simulink model "servoHbridgePraxisbericht"  (R2015a)
settings: Solver=ode23tb  StartTime=0.0  StopTime=1  MaxStep=0.02  RelTol=1e-4
model workspace (MATLAB code in the model file):
  | m_Kt=1.8; % Torque constant
values from neighbouring files (symbols this model uses):
  A = zeros(SYMPACLEN, SYMPACLEN)    [InputMatFramer.m]    (also in InputMatFramerAbgespeckt.m = zeros(10, 10); OUT_OF_MEMORY.m; TIPS_TRICKS.m = { sqrt(10*(rand(2,10)-0.5)), [sqrt(10*(rand(2,10)-0.5)) sqrt; UngarischeMethode.m = [[1 2 9 8];[3 0 3 2];[7 4 1 4];[4 2 7 7]])
  N = (2^16-1)    (= 65535)    [AD_DA.m]    (also in AFB_polynom_interpol.m = 8; UMTSb.m = 160000)
undefined symbols (not defined in the file or in its folder): sigbuilder_block
libraries: powerlib x19
Description:
  | Copyright 2008-2015 The MathWorks, Inc.
settings Model: CovSFcnEnable=off  Creator=MathWorks  LastModifiedBy=mainster
settings DataIOCC: SignalLoggingSaveFormat=ModelDataLogs
settings OptimizationCC: ExpressionDepthLimit=2147483647  InitFltsAndDblsToZero=on
settings DebuggingCC: SaveWithParameterizedLinksMsg=none  UnderspecifiedInitializationDetection=Classic  MergeDetectMultiDrivingBlocksExec=none  SignalResolutionControl=TryResolveAllWithWarning  MaxConsecutiveZCsMsg=warning  SolverPrmCheckMsg=warning  MultiTaskDSMMsg=warning  MultiTaskCondExecSysMsg=none  FcnCallInpInsideContextMsg=UseLocalSettings  StateNameClashWarn=warning
settings GRTTargetCC: TargetFcnLib=ansi_tfl_tmw.mat  CombineOutputUpdateFcns=off  GRTInterface=on

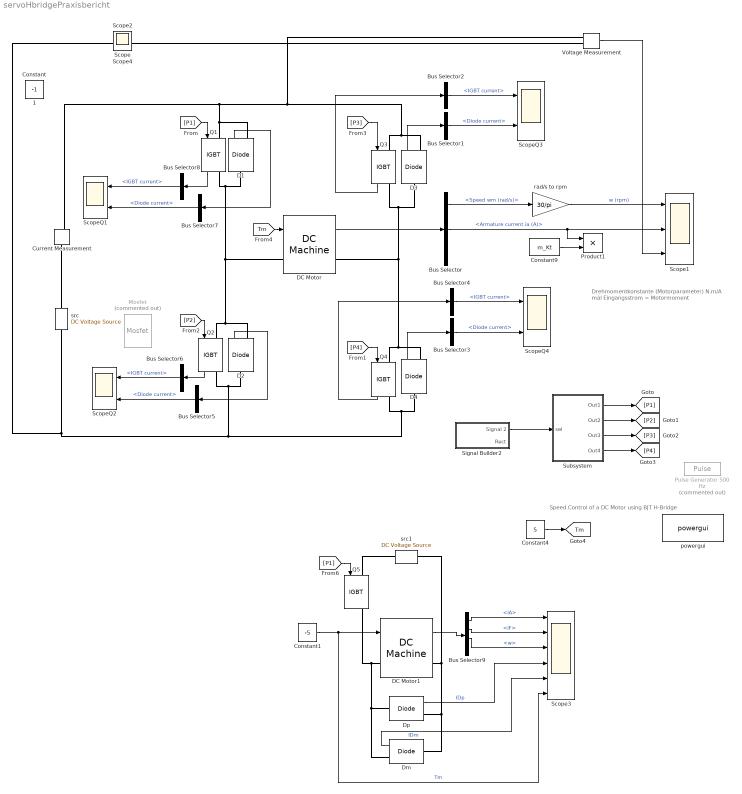
== system servoHbridgePraxisbericht ==
  note: Drehmomentkonstante (Motorparameter) N.m/A
      | mal Eingangsstrom = Motormoment
  note: Speed Control of a DC Motor using BJT H-Bridge
  Bus Selector : BusSelector  OutputSignals=Speed wm (rad/s),Armature current ia (A),Electrical torque Te (n m)
  Bus Selector{1,3,5,7} (4 alike) : BusSelector  OutputSignals=Diode current
  Bus Selector{2,4,6,8} (4 alike) : BusSelector  OutputSignals=IGBT current
  Bus Selector9 : BusSelector  OutputSignals=iA,iF,w,Te
  Constant1 : Constant  Value=-5
  Constant4 : Constant  Value=5
  Constant9 : Constant  Value=m_Kt
  Current Measurement : powerlib/Measurements/Current Measurement  PhasorSimulation=off  OutputType=Complex  PSBequivalent=0
  D{1..4} (4 alike) : powerlib/Power Electronics/Diode  Ron=0.001  Lon=0  Vf=0.8  IC=0  UseSnubber=off  Rs=inf  Cs=0  Measurements=on
  DC Motor : powerlib/Machines/DC Machine  PresetModel=No  MechanicalLoad=Torque TL  FieldType=Permanent magnet  ShowDetailedParameters=on  MeasurementBus=off  RLa=[1 10e-3]  RLf=[281.2 156]  Laf=0.9483  MachineConstant=Torque constant (N.m/A)  Ke=1.8  Kt=m_Kt  J=0.02215  Bm=0.002953  Tf=0.5161  w0=0.001  Ifinit=1.06647707074298  TsPowergui=0  TsBlock=-1
  DC Motor1 : powerlib/Machines/DC Machine  PresetModel=No  MechanicalLoad=Torque TL  FieldType=Permanent magnet  ShowDetailedParameters=on  MeasurementBus=on  RLa=[10 10e-3]  RLf=[281.2 156]  Laf=0.9483  MachineConstant=Torque constant (N.m/A)  Ke=1.8  Kt=m_Kt  J=0.02215  Bm=0.002953  Tf=0.5161  w0=0.001  Ifinit=1  TsPowergui=0  TsBlock=-1
  Dm : powerlib/Power Electronics/Diode  Ron=0.001  Lon=0  Vf=0.8  IC=0  UseSnubber=off  Rs=inf  Cs=0  Measurements=on
  Dp : powerlib/Power Electronics/Diode  Ron=0.001  Lon=0  Vf=0.8  IC=0  UseSnubber=off  Rs=inf  Cs=0  Measurements=on
  Mosfet : powerlib/Power Electronics/Mosfet  Commented=on  Ron=0.1  Lon=0  Rd=0.01  Vfd=.7  IC=0  Rs=1e5  Cs=inf  Measurements=on
  Product1 : Product  RndMeth=Zero
  Pulse Generator 500 Hz : DiscretePulseGenerator  Commented=on  PulseType=Time based  Period=2e-3  PulseWidth=75
  Q{1..5} (5 alike) : powerlib/Power Electronics/IGBT  Ron=0.001  Lon=0  Vf=1  Tf=0  Tt=0  IC=0  Rs=1e5  Cs=inf  Measurements=on
  Scope1 : Scope  NumInputPorts=3
      settings: TimeRange=1  YMin=-100~-10~-20  YMax=100~20~40
  Scope3 : Scope  NumInputPorts=6
      settings: TimeRange=1  YMin=0~-1~-15~-2000~-10~4  YMax=4~1~5~6000~5~6  SaveName=ScopeData7
  ScopeQ{1..4} (4 alike) : Scope  NumInputPorts=2
      ScopeQ1 settings: TimeRange=1  YMin=0~-1  YMax=15~1  SaveName=ScopeData4
      ScopeQ2 settings: TimeRange=1  YMin=0~0  YMax=4~4  SaveName=ScopeData3
      ScopeQ3 settings: TimeRange=1  YMin=0~0  YMax=4~4
      ScopeQ4 settings: TimeRange=1  YMin=0~-1  YMax=15~1  SaveName=ScopeData2
  Signal Builder2 : Subsystem  Tag=STV Subsys  LoadFcn=sigbuilder_block('load');  StartFcn=sigbuilder_block('start');  StopFcn=sigbuilder_block('stop');  ClipboardFcn=sigbuilder_block('clipboard');  mask(Sigbuilder block){}
      mask help: Simulink:masks:SigbuilderBlock_MD
      mask init:
      | if ~strcmp(get_param(bdroot(gcbh),'SimulationStatus'),'stopped') tuvar = sigbuilder_block('maskInit'); end
      settings: CopyFcn=sigbuilder_block('copy');  DeleteFcn=sigbuilder_block('delete');  ModelCloseFcn=sigbuilder_block('modelClose');  PreSaveFcn=sigbuilder_block('preSave');  PauseFcn=sigbuilder_block('pause');  ContinueFcn=sigbuilder_block('continue');  NameChangeFcn=sigbuilder_block('namechange');  OpenFcn=sigbuilder_block('open',[437.6 199.2 550.4 400 ]);  CloseFcn=sigbuilder_block('close');
      mask Display: plot(0, 0, 100, 100,[2, 2, 32, 32, 2], [68, 8, 8, 68, 68],[32, 2], [38, 38], [32, 19, 2],[53, 60, 44], [32, 17, 17, 2],[16, 16, 31, 31]);txt = getActiveGroup(gcbh);text(2, 100, txt,'verticalAlignment', 'top');
  Subsystem : Subsystem
  Voltage Measurement : powerlib/Measurements/Voltage Measurement  PhasorSimulation=off  OutputType=Complex  PSBequivalent=0
  powergui : powerlib/powergui  SimulationMode=Continuous  SolverType=Tustin  SampleTime=20e-6  frequency=60  SPID=on  DisableSnubberDevices=on  DisableRonSwitches=off  DisableVfSwitches=off  SwTol=0  DisplayEquations=off  Interpol=off  methode=off  Ts=0  FunctionMessages=off  echomessages=off  HookPort=off  EnableUseOfTLC=off  x0status=blocks  frequencyindice=0  Pbase=100e6  ErrMax=1e-4  Iterations=50  UnitsV=kV  UnitsW=MW  buscounter=0  RestoreLinks=warning  ResistiveCurrentMeasurement=off  Frange=[0:2:500]  Ylog=off  Xlog=on  ShowGrid=off  save=off  variable=ZData  structure=0  ZoomFFT=on  StartTime=0.0  cycles=1  DisplayStyle=1  fundamental=60  FreqAxis=off  MaxFrequency=1000  frequencyindicesteady=1  RmsSteady=1  display=off
  rad/s to rpm : Gain  Gain=30/pi
  src : powerlib/Electrical Sources/DC Voltage Source  Amplitude=12  Measurements=Voltage
      settings: AttributesFormatString=%<Amplitude>V
  src1 : powerlib/Electrical Sources/DC Voltage Source  Amplitude=12  Measurements=Voltage
      settings: AttributesFormatString=%<Amplitude>V
  1 : Constant  IOType=siggen
  Constant : Constant  IOType=siggen  Value=-1
  Scope : Scope  NumInputPorts=5
      settings: YMin=-0.1~-0.1~-0.1~-0.1~-5  YMax=1.1~1.1~1.1~1.1~5  SaveName=ScopeData5
  Scope2 : Scope  NumInputPorts=2
      settings: YMin=-5~-5  YMax=5~5  SaveName=ScopeData6
  Scope4 : Scope
      settings: TimeRange=1  YMin=0  YMax=6000  SaveName=ScopeData8
  tag scope: Tm=global
  wires:
  Bus Selector/2 -> Product1/1, Scope1/2  "<Armature current ia (A)>"
  rad/s to rpm/1 -> Scope1/1  "w (rpm)"
  Bus Selector/1 -> rad/s to rpm/1  "<Speed wm (rad/s)>"
  DC Motor/1 -> Bus Selector/1
  [P1] -> Q1/1
  [P4] -> Q4/1
  [P2] -> Q2/1
  [P3] -> Q3/1
  D3/1 -> Bus Selector1/1
  Q3/1 -> Bus Selector2/1
  Bus Selector2/1 -> ScopeQ3/1  "<IGBT current>"
  Bus Selector1/1 -> ScopeQ3/2  "<Diode current>"
  [Tm] -> DC Motor/1
  Constant4/1 -> [Tm]
  Constant9/1 -> Product1/2
  Bus Selector4/1 -> ScopeQ4/1  "<IGBT current>"
  Bus Selector3/1 -> ScopeQ4/2  "<Diode current>"
  Subsystem/1(Out1) -> [P1]
  Subsystem/2(Out2) -> [P2]
  Subsystem/3(Out3) -> [P3]
  Subsystem/4(Out4) -> [P4]
  D4/1 -> Bus Selector3/1
  Q4/1 -> Bus Selector4/1
  Bus Selector6/1 -> ScopeQ2/1  "<IGBT current>"
  Bus Selector5/1 -> ScopeQ2/2  "<Diode current>"
  Q2/1 -> Bus Selector6/1
  D2/1 -> Bus Selector5/1
  Bus Selector8/1 -> ScopeQ1/1  "<IGBT current>"
  Bus Selector7/1 -> ScopeQ1/2  "<Diode current>"
  Q1/1 -> Bus Selector8/1
  D1/1 -> Bus Selector7/1
  Signal Builder2/1(Signal 2) -> Subsystem/1(sel)
  Voltage Measurement/1 -> Scope1/3
  DC Motor1/1 -> Bus Selector9/1
  Bus Selector9/1 -> Scope3/1  "<iA>"
  Bus Selector9/3 -> Scope3/3  "<w>"
  Bus Selector9/2 -> Scope3/2  "<iF>"
  Dp/1 -> Scope3/4  "IDp"
  Dm/1 -> Scope3/5  "IDm"
  Constant1/1 -> Scope3/6, DC Motor1/1  "Tm"
  [P1] -> Q5/1
  connections:
  DC Motor/LConn1 -- D1/LConn1 -- Q1/RConn1 -- Q2/LConn1 -- D2/RConn1
  Q4/RConn1 -- D4/LConn1 -- Voltage Measurement/LConn2 -- src/LConn1 -- Q2/RConn1 -- D2/LConn1
  DC Motor/RConn1 -- Q4/LConn1 -- D4/RConn1 -- Q3/RConn1 -- D3/LConn1
  D1/RConn1 -- Q1/LConn1 -- Current Measurement/RConn1 -- Voltage Measurement/LConn1 -- Q3/LConn1 -- D3/RConn1
  Current Measurement/LConn1 -- src/RConn1
  DC Motor1/LConn1 -- Q5/RConn1 -- Dm/RConn1 -- Dp/LConn1
  Dp/RConn1 -- src1/LConn1 -- DC Motor1/RConn1 -- Dm/LConn1
  Q5/LConn1 -- src1/RConn1

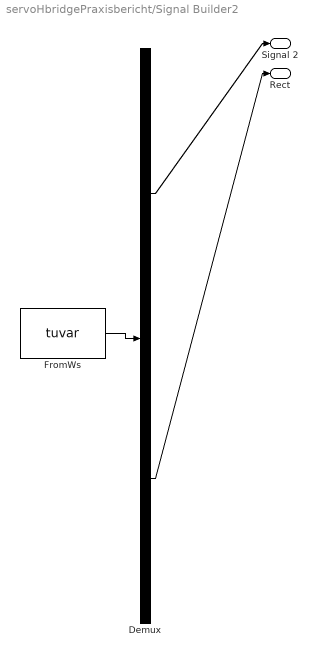
== system servoHbridgePraxisbericht/Signal Builder2 ==
  Demux : Demux  Tag=STV Demux  Outputs=2
  FromWs : FromWorkspace  Tag=STV FromWs  VariableName=tuvar  SampleTime=0
      SigBuilderData=|
      | common.afterFinalStr = 'Extrapolate'
      | common.sampleTime = 0
      | dataSet.timeRange = [0 1]
      | dataSet.name = 'Group 1'
      | sbobj.Groups.Name = 'Group 1'
      | sbobj.Groups.Signals(1).Name = 'Signal 2'
      | sbobj.Groups.Signals(1).XData = [0 0.1 0.106 0.3 0.496 0.5 0.694 0.7 0.8 0.9 1]
      | sbobj.Groups.Signals(1).YData = [1 1 1 1 1 2 2 3 3 3 3]
      | sbobj.Groups.Signals(2).Name = 'Rect'
      | sbobj.Groups.Signals(2).XData = [0 0.25 0.25 0.5 0.5 0.75 0.75 1]
      | sbobj.Groups.Signals(2).YData = [0 0 0.9 0.9 0 0 -1 -1]
      | sbobj.Groups.TimeRange = [0 1]
  Signal 2 : Outport  Tag=STV Outport
  Rect : Outport  Tag=STV Outport  Port=2
  wires:
  FromWs/1 -> Demux/1
  Demux/1 -> Signal 2/1
  Demux/2 -> Rect/1

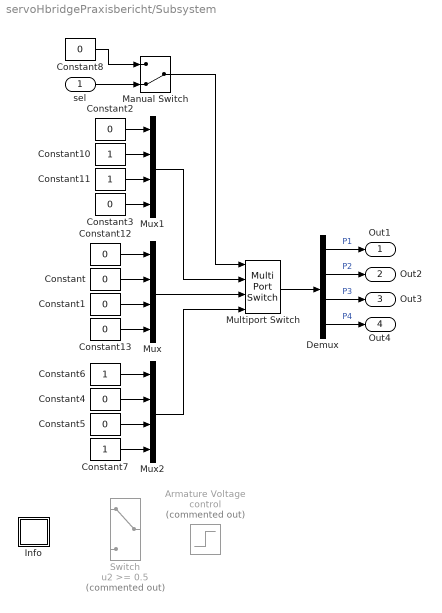
== system servoHbridgePraxisbericht/Subsystem ==
  sel : Inport
  Armature Voltage control : Step  Commented=on  Time=0.5  SampleTime=0
  Constant{,1..5,8,12..13} (9 alike) : Constant  Value=0
  Constant{6..7,10..11} (4 alike) : Constant
  Demux : Demux
  Info : Subsystem
      settings: OpenFcn=showdemo(bdroot(gcb))
      mask Display: disp('?')
  Manual Switch : ManualSwitch  CurrentSetting=0
  Multiport Switch : MultiPortSwitch
  Mux : Mux
  Mux1 : Mux
  Mux2 : Mux
  Switch : Switch  Commented=on  Threshold=0.5
  Out1 : Outport
  Out2 : Outport  Port=2
  Out3 : Outport  Port=3
  Out4 : Outport  Port=4
  wires:
  Demux/2 -> Out2/1  "P2"
  Demux/3 -> Out3/1  "P3"
  Constant12/1 -> Mux/1
  Constant10/1 -> Mux1/2
  Constant11/1 -> Mux1/3
  Demux/4 -> Out4/1  "P4"
  Demux/1 -> Out1/1  "P1"
  Constant13/1 -> Mux/4
  Constant2/1 -> Mux1/1
  Multiport Switch/1 -> Demux/1
  Constant1/1 -> Mux/3
  Constant/1 -> Mux/2
  Mux/1 -> Multiport Switch/3
  Constant3/1 -> Mux1/4
  Mux1/1 -> Multiport Switch/2
  Constant6/1 -> Mux2/1
  Constant7/1 -> Mux2/4
  Constant5/1 -> Mux2/3
  Constant4/1 -> Mux2/2
  Mux2/1 -> Multiport Switch/4
  Manual Switch/1 -> Multiport Switch/1
  sel/1 -> Manual Switch/2
  Constant8/1 -> Manual Switch/1

== system servoHbridgePraxisbericht/Subsystem/Info ==
